simulink model "dsp48_firs_tb"  (Simulink 7.0)
settings: Solver=ode45  StartTime=0.0  StopTime=200  RelTol=1e-3
PreLoadFcn:
  | fir_setup_v1
StartFcn:
  | fir_setup_v1
undefined symbols (not defined in the file): A, B, C, coef, P, PCIN
libraries: xbsIndex_r4 x229, simulink x10, xbsCopyrightNotice_r4 x1, dspsrcs4 x1
(part 3 of 3)

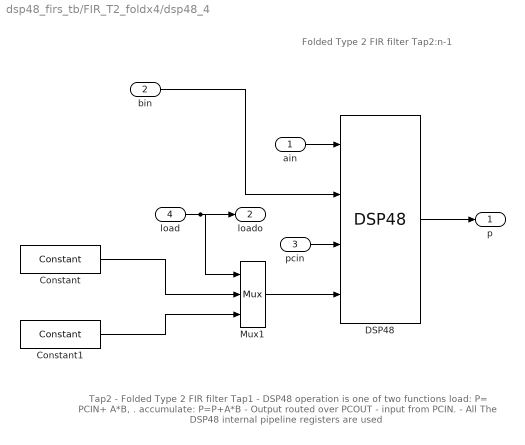
== system dsp48_firs_tb/FIR_T2_foldx4/dsp48_4 ==
  note: Folded Type 2 FIR filter Tap2:n-1
  note: Tap2 - Folded Type 2 FIR filter Tap1
      | - DSP48 operation is one of two functions
      |   load:  P= PCIN+ A*B, .
      |   accumulate: P=P+A*B
      | - Output routed over PCOUT
      | - input from PCIN.
      | - All The DSP48 internal pipeline registers are used
  ain : Inport  OutDataType=sfix(16)  OutScaling=2^0
  bin : Inport  Port=2  OutDataType=sfix(16)  OutScaling=2^0
  pcin : Inport  Port=3  OutDataType=sfix(16)  OutScaling=2^0
  load : Inport  Port=4  OutDataType=sfix(16)  OutScaling=2^0
  Constant : xbsIndex_r4/Constant  arith_type=DSP48 Instruction  const=1  n_bits=1  bin_pt=0  explicit_period=off  period=1  equ=P=P+(A*B)  opselect=P + A*B  inp2=PCIN>>17  opr=+  inp1=P  carry=CIN  dbl_ovrd=off  block_type=constant
      settings: block_version=VER_STRING_GOES_HERE
  Constant1 : xbsIndex_r4/Constant  arith_type=DSP48 Instruction  const=1  n_bits=1  bin_pt=0  explicit_period=off  period=1  equ=P=PCIN+(A*B)  opselect=PCIN + A*B  inp2=PCIN>>17  opr=+  inp1=P  carry=CIN  dbl_ovrd=off  block_type=constant
      settings: block_version=VER_STRING_GOES_HERE
  DSP48 : xbsIndex_r4/DSP48  use_b=Direct from B Port  use_op=on  use_creg=off  use_pcin=on  use_pcout=off  use_bcout=off  rst_all=off  en_all=off  pipeline_a=1  pipeline_b=1  pipeline_c=on  pipeline_p=on  pipeline_mult=on  pipeline_opmode=on  pipeline_sub=on  pipeline_carryin=on  pipeline_carryinsel=on  rst_a=off  rst_b=off  rst_c=off  rst_mult=off  rst_p=off  rst_carry_in=off  rst_ctrl=off  en_a=off  en_b=off  en_c=off  en_mult=off  en_p=off  en_carry_in=off  en_ctrl=off  dbl_ovrd=off  use_synth_model=off  xl_useadderonly=off  block_type=dsp48
      settings: xl_use_area=on  xl_area=[0, 0, 0, 0, 0, 0, 0]  block_version=VER_STRING_GOES_HERE
  Mux1 : xbsIndex_r4/Mux  inputs=2  en=off  latency=0  precision=Full  arith_type=Unsigned  n_bits=48  bin_pt=0  quantization=Truncate  overflow=Wrap  dbl_ovrd=off  block_type=mux
      settings: xl_area=[0, 0, 0, 0, 0, 0, 0]  block_version=VER_STRING_GOES_HERE
  p : Outport  OutDataType=sfix(16)  OutScaling=2^0
  loado : Outport  Port=2  OutDataType=sfix(16)  OutScaling=2^0
  wires:
  bin/1 -> DSP48/2
  ain/1 -> DSP48/1
  Constant1/1 -> Mux1/3
  Constant/1 -> Mux1/2
  load/1 -> loado/1, Mux1/1
  DSP48/1 -> p/1
  pcin/1 -> DSP48/3
  Mux1/1 -> DSP48/4

== system dsp48_firs_tb/FIR_T2x16 /fir_last ==
  note: Tapn- Parallel Type2 FIR filter
      | - DSP48 operation is the  function P=PCIN+ A*B.
      | - Input over PCIN, output is from P
      | - All The DSP48 internal pipeline registers are used
      | - The BCIN-BCOUT cascade is not used
  note: Parallel FIR Type2 Tap #n
  ain : Inport  OutDataType=sfix(16)  OutScaling=2^0
  bin : Inport  Port=2  OutDataType=sfix(16)  OutScaling=2^0
  pcin : Inport  Port=3  OutDataType=sfix(16)  OutScaling=2^0
  Constant1 : xbsIndex_r4/Constant  arith_type=DSP48 Instruction  const=1  n_bits=1  bin_pt=0  explicit_period=off  period=1  equ=P=PCIN+(A*B)  opselect=PCIN + A*B  inp2=PCIN>>17  opr=+  inp1=P  carry=CIN  dbl_ovrd=off  block_type=constant
      settings: block_version=VER_STRING_GOES_HERE
  DSP48 : xbsIndex_r4/DSP48  use_b=Direct from B Port  use_op=on  use_creg=off  use_pcin=on  use_pcout=off  use_bcout=off  rst_all=off  en_all=off  pipeline_a=1  pipeline_b=1  pipeline_c=on  pipeline_p=on  pipeline_mult=on  pipeline_opmode=on  pipeline_sub=on  pipeline_carryin=on  pipeline_carryinsel=on  rst_a=off  rst_b=off  rst_c=off  rst_mult=off  rst_p=off  rst_carry_in=off  rst_ctrl=off  en_a=off  en_b=off  en_c=off  en_mult=off  en_p=off  en_carry_in=off  en_ctrl=off  dbl_ovrd=off  use_synth_model=off  xl_useadderonly=off  block_type=dsp48
      settings: xl_use_area=on  xl_area=[0, 0, 0, 0, 0, 0, 0]  block_version=VER_STRING_GOES_HERE
  p : Outport  OutDataType=sfix(16)  OutScaling=2^0
  wires:
  bin/1 -> DSP48/2
  DSP48/1 -> p/1
  ain/1 -> DSP48/1
  pcin/1 -> DSP48/3
  Constant1/1 -> DSP48/4

== system dsp48_firs_tb/FIR_T2x16 /fir_next1 ==
  note: Tap2,n-1 - Parallel Type2 FIR filter
      | - DSP48 operation is the  function P=PCIN+ A*B.
      | - Input and Output routed over PCIN-PCOUT.
      | - All The DSP48 internal pipeline registers are used
      | - The BCIN-BCOUT cascade is not used
  note: Parallel FIR Type2 Tap #2:n-1
  ain : Inport  OutDataType=sfix(16)  OutScaling=2^0
  bin : Inport  Port=2  OutDataType=sfix(16)  OutScaling=2^0
  pcin : Inport  Port=3  OutDataType=sfix(16)  OutScaling=2^0
  Constant1 : xbsIndex_r4/Constant  arith_type=DSP48 Instruction  const=1  n_bits=1  bin_pt=0  explicit_period=off  period=1  equ=P=PCIN+(A*B)  opselect=PCIN + A*B  inp2=PCIN>>17  opr=+  inp1=P  carry=CIN  dbl_ovrd=off  block_type=constant
      settings: block_version=VER_STRING_GOES_HERE
  DSP48 : xbsIndex_r4/DSP48  use_b=Direct from B Port  use_op=on  use_creg=off  use_pcin=on  use_pcout=on  use_bcout=off  rst_all=off  en_all=off  pipeline_a=1  pipeline_b=1  pipeline_c=on  pipeline_p=on  pipeline_mult=on  pipeline_opmode=on  pipeline_sub=on  pipeline_carryin=on  pipeline_carryinsel=on  rst_a=off  rst_b=off  rst_c=off  rst_mult=off  rst_p=off  rst_carry_in=off  rst_ctrl=off  en_a=off  en_b=off  en_c=off  en_mult=off  en_p=off  en_carry_in=off  en_ctrl=off  dbl_ovrd=off  use_synth_model=off  xl_useadderonly=off  block_type=dsp48
      settings: xl_use_area=on  xl_area=[0, 0, 0, 0, 0, 0, 0]  block_version=VER_STRING_GOES_HERE
  Terminator1 : Terminator
  bout : Outport  OutDataType=sfix(16)  OutScaling=2^0
  pcout : Outport  Port=2  OutDataType=sfix(16)  OutScaling=2^0
  wires:
  bin/1 -> bout/1, DSP48/2
  ain/1 -> DSP48/1
  DSP48/2 -> pcout/1
  DSP48/1 -> Terminator1/1
  pcin/1 -> DSP48/3
  Constant1/1 -> DSP48/4

== system dsp48_firs_tb/FIR_T2x16 /fir_next10 ==
  note: Parallel FIR Type2 Tap #2:n-1
  note: Tap2,n-1 - Parallel Type2 FIR filter
      | - DSP48 operation is the  function P=PCIN+ A*B.
      | - Input and Output routed over PCIN-PCOUT.
      | - All The DSP48 internal pipeline registers are used
      | - The BCIN-BCOUT cascade is not used
  ain : Inport  OutDataType=sfix(16)  OutScaling=2^0
  bin : Inport  Port=2  OutDataType=sfix(16)  OutScaling=2^0
  pcin : Inport  Port=3  OutDataType=sfix(16)  OutScaling=2^0
  Constant1 : xbsIndex_r4/Constant  arith_type=DSP48 Instruction  const=1  n_bits=1  bin_pt=0  explicit_period=off  period=1  equ=P=PCIN+(A*B)  opselect=PCIN + A*B  inp2=PCIN>>17  opr=+  inp1=P  carry=CIN  dbl_ovrd=off  block_type=constant
      settings: block_version=VER_STRING_GOES_HERE
  DSP48 : xbsIndex_r4/DSP48  use_b=Direct from B Port  use_op=on  use_creg=off  use_pcin=on  use_pcout=on  use_bcout=off  rst_all=off  en_all=off  pipeline_a=1  pipeline_b=1  pipeline_c=on  pipeline_p=on  pipeline_mult=on  pipeline_opmode=on  pipeline_sub=on  pipeline_carryin=on  pipeline_carryinsel=on  rst_a=off  rst_b=off  rst_c=off  rst_mult=off  rst_p=off  rst_carry_in=off  rst_ctrl=off  en_a=off  en_b=off  en_c=off  en_mult=off  en_p=off  en_carry_in=off  en_ctrl=off  dbl_ovrd=off  use_synth_model=off  xl_useadderonly=off  block_type=dsp48
      settings: xl_use_area=on  xl_area=[0, 0, 0, 0, 0, 0, 0]  block_version=VER_STRING_GOES_HERE
  Terminator1 : Terminator
  bout : Outport  OutDataType=sfix(16)  OutScaling=2^0
  pcout : Outport  Port=2  OutDataType=sfix(16)  OutScaling=2^0
  wires:
  Constant1/1 -> DSP48/4
  pcin/1 -> DSP48/3
  DSP48/1 -> Terminator1/1
  DSP48/2 -> pcout/1
  ain/1 -> DSP48/1
  bin/1 -> DSP48/2, bout/1

== system dsp48_firs_tb/FIR_T2x16 /fir_next11 ==
  note: Tap2,n-1 - Parallel Type2 FIR filter
      | - DSP48 operation is the  function P=PCIN+ A*B.
      | - Input and Output routed over PCIN-PCOUT.
      | - All The DSP48 internal pipeline registers are used
      | - The BCIN-BCOUT cascade is not used
  note: Parallel FIR Type2 Tap #2:n-1
  ain : Inport  OutDataType=sfix(16)  OutScaling=2^0
  bin : Inport  Port=2  OutDataType=sfix(16)  OutScaling=2^0
  pcin : Inport  Port=3  OutDataType=sfix(16)  OutScaling=2^0
  Constant1 : xbsIndex_r4/Constant  arith_type=DSP48 Instruction  const=1  n_bits=1  bin_pt=0  explicit_period=off  period=1  equ=P=PCIN+(A*B)  opselect=PCIN + A*B  inp2=PCIN>>17  opr=+  inp1=P  carry=CIN  dbl_ovrd=off  block_type=constant
      settings: block_version=VER_STRING_GOES_HERE
  DSP48 : xbsIndex_r4/DSP48  use_b=Direct from B Port  use_op=on  use_creg=off  use_pcin=on  use_pcout=on  use_bcout=off  rst_all=off  en_all=off  pipeline_a=1  pipeline_b=1  pipeline_c=on  pipeline_p=on  pipeline_mult=on  pipeline_opmode=on  pipeline_sub=on  pipeline_carryin=on  pipeline_carryinsel=on  rst_a=off  rst_b=off  rst_c=off  rst_mult=off  rst_p=off  rst_carry_in=off  rst_ctrl=off  en_a=off  en_b=off  en_c=off  en_mult=off  en_p=off  en_carry_in=off  en_ctrl=off  dbl_ovrd=off  use_synth_model=off  xl_useadderonly=off  block_type=dsp48
      settings: xl_use_area=on  xl_area=[0, 0, 0, 0, 0, 0, 0]  block_version=VER_STRING_GOES_HERE
  Terminator1 : Terminator
  bout : Outport  OutDataType=sfix(16)  OutScaling=2^0
  pcout : Outport  Port=2  OutDataType=sfix(16)  OutScaling=2^0
  wires:
  bin/1 -> bout/1, DSP48/2
  ain/1 -> DSP48/1
  DSP48/2 -> pcout/1
  DSP48/1 -> Terminator1/1
  pcin/1 -> DSP48/3
  Constant1/1 -> DSP48/4

== system dsp48_firs_tb/FIR_T2x16 /fir_next12 ==
  note: Parallel FIR Type2 Tap #2:n-1
  note: Tap2,n-1 - Parallel Type2 FIR filter
      | - DSP48 operation is the  function P=PCIN+ A*B.
      | - Input and Output routed over PCIN-PCOUT.
      | - All The DSP48 internal pipeline registers are used
      | - The BCIN-BCOUT cascade is not used
  ain : Inport  OutDataType=sfix(16)  OutScaling=2^0
  bin : Inport  Port=2  OutDataType=sfix(16)  OutScaling=2^0
  pcin : Inport  Port=3  OutDataType=sfix(16)  OutScaling=2^0
  Constant1 : xbsIndex_r4/Constant  arith_type=DSP48 Instruction  const=1  n_bits=1  bin_pt=0  explicit_period=off  period=1  equ=P=PCIN+(A*B)  opselect=PCIN + A*B  inp2=PCIN>>17  opr=+  inp1=P  carry=CIN  dbl_ovrd=off  block_type=constant
      settings: block_version=VER_STRING_GOES_HERE
  DSP48 : xbsIndex_r4/DSP48  use_b=Direct from B Port  use_op=on  use_creg=off  use_pcin=on  use_pcout=on  use_bcout=off  rst_all=off  en_all=off  pipeline_a=1  pipeline_b=1  pipeline_c=on  pipeline_p=on  pipeline_mult=on  pipeline_opmode=on  pipeline_sub=on  pipeline_carryin=on  pipeline_carryinsel=on  rst_a=off  rst_b=off  rst_c=off  rst_mult=off  rst_p=off  rst_carry_in=off  rst_ctrl=off  en_a=off  en_b=off  en_c=off  en_mult=off  en_p=off  en_carry_in=off  en_ctrl=off  dbl_ovrd=off  use_synth_model=off  xl_useadderonly=off  block_type=dsp48
      settings: xl_use_area=on  xl_area=[0, 0, 0, 0, 0, 0, 0]  block_version=VER_STRING_GOES_HERE
  Terminator1 : Terminator
  bout : Outport  OutDataType=sfix(16)  OutScaling=2^0
  pcout : Outport  Port=2  OutDataType=sfix(16)  OutScaling=2^0
  wires:
  Constant1/1 -> DSP48/4
  pcin/1 -> DSP48/3
  DSP48/1 -> Terminator1/1
  DSP48/2 -> pcout/1
  ain/1 -> DSP48/1
  bin/1 -> DSP48/2, bout/1

== system dsp48_firs_tb/FIR_T2x16 /fir_next13 ==
  note: Tap2,n-1 - Parallel Type2 FIR filter
      | - DSP48 operation is the  function P=PCIN+ A*B.
      | - Input and Output routed over PCIN-PCOUT.
      | - All The DSP48 internal pipeline registers are used
      | - The BCIN-BCOUT cascade is not used
  note: Parallel FIR Type2 Tap #2:n-1
  ain : Inport  OutDataType=sfix(16)  OutScaling=2^0
  bin : Inport  Port=2  OutDataType=sfix(16)  OutScaling=2^0
  pcin : Inport  Port=3  OutDataType=sfix(16)  OutScaling=2^0
  Constant1 : xbsIndex_r4/Constant  arith_type=DSP48 Instruction  const=1  n_bits=1  bin_pt=0  explicit_period=off  period=1  equ=P=PCIN+(A*B)  opselect=PCIN + A*B  inp2=PCIN>>17  opr=+  inp1=P  carry=CIN  dbl_ovrd=off  block_type=constant
      settings: block_version=VER_STRING_GOES_HERE
  DSP48 : xbsIndex_r4/DSP48  use_b=Direct from B Port  use_op=on  use_creg=off  use_pcin=on  use_pcout=on  use_bcout=off  rst_all=off  en_all=off  pipeline_a=1  pipeline_b=1  pipeline_c=on  pipeline_p=on  pipeline_mult=on  pipeline_opmode=on  pipeline_sub=on  pipeline_carryin=on  pipeline_carryinsel=on  rst_a=off  rst_b=off  rst_c=off  rst_mult=off  rst_p=off  rst_carry_in=off  rst_ctrl=off  en_a=off  en_b=off  en_c=off  en_mult=off  en_p=off  en_carry_in=off  en_ctrl=off  dbl_ovrd=off  use_synth_model=off  xl_useadderonly=off  block_type=dsp48
      settings: xl_use_area=on  xl_area=[0, 0, 0, 0, 0, 0, 0]  block_version=VER_STRING_GOES_HERE
  Terminator1 : Terminator
  bout : Outport  OutDataType=sfix(16)  OutScaling=2^0
  pcout : Outport  Port=2  OutDataType=sfix(16)  OutScaling=2^0
  wires:
  bin/1 -> bout/1, DSP48/2
  ain/1 -> DSP48/1
  DSP48/2 -> pcout/1
  DSP48/1 -> Terminator1/1
  pcin/1 -> DSP48/3
  Constant1/1 -> DSP48/4

== system dsp48_firs_tb/FIR_T2x16 /fir_next14 ==
  note: Parallel FIR Type2 Tap #2:n-1
  note: Tap2,n-1 - Parallel Type2 FIR filter
      | - DSP48 operation is the  function P=PCIN+ A*B.
      | - Input and Output routed over PCIN-PCOUT.
      | - All The DSP48 internal pipeline registers are used
      | - The BCIN-BCOUT cascade is not used
  ain : Inport  OutDataType=sfix(16)  OutScaling=2^0
  bin : Inport  Port=2  OutDataType=sfix(16)  OutScaling=2^0
  pcin : Inport  Port=3  OutDataType=sfix(16)  OutScaling=2^0
  Constant1 : xbsIndex_r4/Constant  arith_type=DSP48 Instruction  const=1  n_bits=1  bin_pt=0  explicit_period=off  period=1  equ=P=PCIN+(A*B)  opselect=PCIN + A*B  inp2=PCIN>>17  opr=+  inp1=P  carry=CIN  dbl_ovrd=off  block_type=constant
      settings: block_version=VER_STRING_GOES_HERE
  DSP48 : xbsIndex_r4/DSP48  use_b=Direct from B Port  use_op=on  use_creg=off  use_pcin=on  use_pcout=on  use_bcout=off  rst_all=off  en_all=off  pipeline_a=1  pipeline_b=1  pipeline_c=on  pipeline_p=on  pipeline_mult=on  pipeline_opmode=on  pipeline_sub=on  pipeline_carryin=on  pipeline_carryinsel=on  rst_a=off  rst_b=off  rst_c=off  rst_mult=off  rst_p=off  rst_carry_in=off  rst_ctrl=off  en_a=off  en_b=off  en_c=off  en_mult=off  en_p=off  en_carry_in=off  en_ctrl=off  dbl_ovrd=off  use_synth_model=off  xl_useadderonly=off  block_type=dsp48
      settings: xl_use_area=on  xl_area=[0, 0, 0, 0, 0, 0, 0]  block_version=VER_STRING_GOES_HERE
  Terminator1 : Terminator
  bout : Outport  OutDataType=sfix(16)  OutScaling=2^0
  pcout : Outport  Port=2  OutDataType=sfix(16)  OutScaling=2^0
  wires:
  Constant1/1 -> DSP48/4
  pcin/1 -> DSP48/3
  DSP48/1 -> Terminator1/1
  DSP48/2 -> pcout/1
  ain/1 -> DSP48/1
  bin/1 -> DSP48/2, bout/1

== system dsp48_firs_tb/FIR_T2x16 /fir_next2 ==
  note: Parallel FIR Type2 Tap #2:n-1
  note: Tap2,n-1 - Parallel Type2 FIR filter
      | - DSP48 operation is the  function P=PCIN+ A*B.
      | - Input and Output routed over PCIN-PCOUT.
      | - All The DSP48 internal pipeline registers are used
      | - The BCIN-BCOUT cascade is not used
  ain : Inport  OutDataType=sfix(16)  OutScaling=2^0
  bin : Inport  Port=2  OutDataType=sfix(16)  OutScaling=2^0
  pcin : Inport  Port=3  OutDataType=sfix(16)  OutScaling=2^0
  Constant1 : xbsIndex_r4/Constant  arith_type=DSP48 Instruction  const=1  n_bits=1  bin_pt=0  explicit_period=off  period=1  equ=P=PCIN+(A*B)  opselect=PCIN + A*B  inp2=PCIN>>17  opr=+  inp1=P  carry=CIN  dbl_ovrd=off  block_type=constant
      settings: block_version=VER_STRING_GOES_HERE
  DSP48 : xbsIndex_r4/DSP48  use_b=Direct from B Port  use_op=on  use_creg=off  use_pcin=on  use_pcout=on  use_bcout=off  rst_all=off  en_all=off  pipeline_a=1  pipeline_b=1  pipeline_c=on  pipeline_p=on  pipeline_mult=on  pipeline_opmode=on  pipeline_sub=on  pipeline_carryin=on  pipeline_carryinsel=on  rst_a=off  rst_b=off  rst_c=off  rst_mult=off  rst_p=off  rst_carry_in=off  rst_ctrl=off  en_a=off  en_b=off  en_c=off  en_mult=off  en_p=off  en_carry_in=off  en_ctrl=off  dbl_ovrd=off  use_synth_model=off  xl_useadderonly=off  block_type=dsp48
      settings: xl_use_area=on  xl_area=[0, 0, 0, 0, 0, 0, 0]  block_version=VER_STRING_GOES_HERE
  Terminator1 : Terminator
  bout : Outport  OutDataType=sfix(16)  OutScaling=2^0
  pcout : Outport  Port=2  OutDataType=sfix(16)  OutScaling=2^0
  wires:
  Constant1/1 -> DSP48/4
  pcin/1 -> DSP48/3
  DSP48/1 -> Terminator1/1
  DSP48/2 -> pcout/1
  ain/1 -> DSP48/1
  bin/1 -> DSP48/2, bout/1

== system dsp48_firs_tb/FIR_T2x16 /fir_next3 ==
  note: Tap2,n-1 - Parallel Type2 FIR filter
      | - DSP48 operation is the  function P=PCIN+ A*B.
      | - Input and Output routed over PCIN-PCOUT.
      | - All The DSP48 internal pipeline registers are used
      | - The BCIN-BCOUT cascade is not used
  note: Parallel FIR Type2 Tap #2:n-1
  ain : Inport  OutDataType=sfix(16)  OutScaling=2^0
  bin : Inport  Port=2  OutDataType=sfix(16)  OutScaling=2^0
  pcin : Inport  Port=3  OutDataType=sfix(16)  OutScaling=2^0
  Constant1 : xbsIndex_r4/Constant  arith_type=DSP48 Instruction  const=1  n_bits=1  bin_pt=0  explicit_period=off  period=1  equ=P=PCIN+(A*B)  opselect=PCIN + A*B  inp2=PCIN>>17  opr=+  inp1=P  carry=CIN  dbl_ovrd=off  block_type=constant
      settings: block_version=VER_STRING_GOES_HERE
  DSP48 : xbsIndex_r4/DSP48  use_b=Direct from B Port  use_op=on  use_creg=off  use_pcin=on  use_pcout=on  use_bcout=off  rst_all=off  en_all=off  pipeline_a=1  pipeline_b=1  pipeline_c=on  pipeline_p=on  pipeline_mult=on  pipeline_opmode=on  pipeline_sub=on  pipeline_carryin=on  pipeline_carryinsel=on  rst_a=off  rst_b=off  rst_c=off  rst_mult=off  rst_p=off  rst_carry_in=off  rst_ctrl=off  en_a=off  en_b=off  en_c=off  en_mult=off  en_p=off  en_carry_in=off  en_ctrl=off  dbl_ovrd=off  use_synth_model=off  xl_useadderonly=off  block_type=dsp48
      settings: xl_use_area=on  xl_area=[0, 0, 0, 0, 0, 0, 0]  block_version=VER_STRING_GOES_HERE
  Terminator1 : Terminator
  bout : Outport  OutDataType=sfix(16)  OutScaling=2^0
  pcout : Outport  Port=2  OutDataType=sfix(16)  OutScaling=2^0
  wires:
  bin/1 -> bout/1, DSP48/2
  ain/1 -> DSP48/1
  DSP48/2 -> pcout/1
  DSP48/1 -> Terminator1/1
  pcin/1 -> DSP48/3
  Constant1/1 -> DSP48/4

== system dsp48_firs_tb/FIR_T2x16 /fir_next4 ==
  note: Parallel FIR Type2 Tap #2:n-1
  note: Tap2,n-1 - Parallel Type2 FIR filter
      | - DSP48 operation is the  function P=PCIN+ A*B.
      | - Input and Output routed over PCIN-PCOUT.
      | - All The DSP48 internal pipeline registers are used
      | - The BCIN-BCOUT cascade is not used
  ain : Inport  OutDataType=sfix(16)  OutScaling=2^0
  bin : Inport  Port=2  OutDataType=sfix(16)  OutScaling=2^0
  pcin : Inport  Port=3  OutDataType=sfix(16)  OutScaling=2^0
  Constant1 : xbsIndex_r4/Constant  arith_type=DSP48 Instruction  const=1  n_bits=1  bin_pt=0  explicit_period=off  period=1  equ=P=PCIN+(A*B)  opselect=PCIN + A*B  inp2=PCIN>>17  opr=+  inp1=P  carry=CIN  dbl_ovrd=off  block_type=constant
      settings: block_version=VER_STRING_GOES_HERE
  DSP48 : xbsIndex_r4/DSP48  use_b=Direct from B Port  use_op=on  use_creg=off  use_pcin=on  use_pcout=on  use_bcout=off  rst_all=off  en_all=off  pipeline_a=1  pipeline_b=1  pipeline_c=on  pipeline_p=on  pipeline_mult=on  pipeline_opmode=on  pipeline_sub=on  pipeline_carryin=on  pipeline_carryinsel=on  rst_a=off  rst_b=off  rst_c=off  rst_mult=off  rst_p=off  rst_carry_in=off  rst_ctrl=off  en_a=off  en_b=off  en_c=off  en_mult=off  en_p=off  en_carry_in=off  en_ctrl=off  dbl_ovrd=off  use_synth_model=off  xl_useadderonly=off  block_type=dsp48
      settings: xl_use_area=on  xl_area=[0, 0, 0, 0, 0, 0, 0]  block_version=VER_STRING_GOES_HERE
  Terminator1 : Terminator
  bout : Outport  OutDataType=sfix(16)  OutScaling=2^0
  pcout : Outport  Port=2  OutDataType=sfix(16)  OutScaling=2^0
  wires:
  Constant1/1 -> DSP48/4
  pcin/1 -> DSP48/3
  DSP48/1 -> Terminator1/1
  DSP48/2 -> pcout/1
  ain/1 -> DSP48/1
  bin/1 -> DSP48/2, bout/1

== system dsp48_firs_tb/FIR_T2x16 /fir_next5 ==
  note: Tap2,n-1 - Parallel Type2 FIR filter
      | - DSP48 operation is the  function P=PCIN+ A*B.
      | - Input and Output routed over PCIN-PCOUT.
      | - All The DSP48 internal pipeline registers are used
      | - The BCIN-BCOUT cascade is not used
  note: Parallel FIR Type2 Tap #2:n-1
  ain : Inport  OutDataType=sfix(16)  OutScaling=2^0
  bin : Inport  Port=2  OutDataType=sfix(16)  OutScaling=2^0
  pcin : Inport  Port=3  OutDataType=sfix(16)  OutScaling=2^0
  Constant1 : xbsIndex_r4/Constant  arith_type=DSP48 Instruction  const=1  n_bits=1  bin_pt=0  explicit_period=off  period=1  equ=P=PCIN+(A*B)  opselect=PCIN + A*B  inp2=PCIN>>17  opr=+  inp1=P  carry=CIN  dbl_ovrd=off  block_type=constant
      settings: block_version=VER_STRING_GOES_HERE
  DSP48 : xbsIndex_r4/DSP48  use_b=Direct from B Port  use_op=on  use_creg=off  use_pcin=on  use_pcout=on  use_bcout=off  rst_all=off  en_all=off  pipeline_a=1  pipeline_b=1  pipeline_c=on  pipeline_p=on  pipeline_mult=on  pipeline_opmode=on  pipeline_sub=on  pipeline_carryin=on  pipeline_carryinsel=on  rst_a=off  rst_b=off  rst_c=off  rst_mult=off  rst_p=off  rst_carry_in=off  rst_ctrl=off  en_a=off  en_b=off  en_c=off  en_mult=off  en_p=off  en_carry_in=off  en_ctrl=off  dbl_ovrd=off  use_synth_model=off  xl_useadderonly=off  block_type=dsp48
      settings: xl_use_area=on  xl_area=[0, 0, 0, 0, 0, 0, 0]  block_version=VER_STRING_GOES_HERE
  Terminator1 : Terminator
  bout : Outport  OutDataType=sfix(16)  OutScaling=2^0
  pcout : Outport  Port=2  OutDataType=sfix(16)  OutScaling=2^0
  wires:
  bin/1 -> bout/1, DSP48/2
  ain/1 -> DSP48/1
  DSP48/2 -> pcout/1
  DSP48/1 -> Terminator1/1
  pcin/1 -> DSP48/3
  Constant1/1 -> DSP48/4

== system dsp48_firs_tb/FIR_T2x16 /fir_next6 ==
  note: Parallel FIR Type2 Tap #2:n-1
  note: Tap2,n-1 - Parallel Type2 FIR filter
      | - DSP48 operation is the  function P=PCIN+ A*B.
      | - Input and Output routed over PCIN-PCOUT.
      | - All The DSP48 internal pipeline registers are used
      | - The BCIN-BCOUT cascade is not used
  ain : Inport  OutDataType=sfix(16)  OutScaling=2^0
  bin : Inport  Port=2  OutDataType=sfix(16)  OutScaling=2^0
  pcin : Inport  Port=3  OutDataType=sfix(16)  OutScaling=2^0
  Constant1 : xbsIndex_r4/Constant  arith_type=DSP48 Instruction  const=1  n_bits=1  bin_pt=0  explicit_period=off  period=1  equ=P=PCIN+(A*B)  opselect=PCIN + A*B  inp2=PCIN>>17  opr=+  inp1=P  carry=CIN  dbl_ovrd=off  block_type=constant
      settings: block_version=VER_STRING_GOES_HERE
  DSP48 : xbsIndex_r4/DSP48  use_b=Direct from B Port  use_op=on  use_creg=off  use_pcin=on  use_pcout=on  use_bcout=off  rst_all=off  en_all=off  pipeline_a=1  pipeline_b=1  pipeline_c=on  pipeline_p=on  pipeline_mult=on  pipeline_opmode=on  pipeline_sub=on  pipeline_carryin=on  pipeline_carryinsel=on  rst_a=off  rst_b=off  rst_c=off  rst_mult=off  rst_p=off  rst_carry_in=off  rst_ctrl=off  en_a=off  en_b=off  en_c=off  en_mult=off  en_p=off  en_carry_in=off  en_ctrl=off  dbl_ovrd=off  use_synth_model=off  xl_useadderonly=off  block_type=dsp48
      settings: xl_use_area=on  xl_area=[0, 0, 0, 0, 0, 0, 0]  block_version=VER_STRING_GOES_HERE
  Terminator1 : Terminator
  bout : Outport  OutDataType=sfix(16)  OutScaling=2^0
  pcout : Outport  Port=2  OutDataType=sfix(16)  OutScaling=2^0
  wires:
  Constant1/1 -> DSP48/4
  pcin/1 -> DSP48/3
  DSP48/1 -> Terminator1/1
  DSP48/2 -> pcout/1
  ain/1 -> DSP48/1
  bin/1 -> DSP48/2, bout/1

== system dsp48_firs_tb/FIR_T2x16 /fir_next7 ==
  note: Tap2,n-1 - Parallel Type2 FIR filter
      | - DSP48 operation is the  function P=PCIN+ A*B.
      | - Input and Output routed over PCIN-PCOUT.
      | - All The DSP48 internal pipeline registers are used
      | - The BCIN-BCOUT cascade is not used
  note: Parallel FIR Type2 Tap #2:n-1
  ain : Inport  OutDataType=sfix(16)  OutScaling=2^0
  bin : Inport  Port=2  OutDataType=sfix(16)  OutScaling=2^0
  pcin : Inport  Port=3  OutDataType=sfix(16)  OutScaling=2^0
  Constant1 : xbsIndex_r4/Constant  arith_type=DSP48 Instruction  const=1  n_bits=1  bin_pt=0  explicit_period=off  period=1  equ=P=PCIN+(A*B)  opselect=PCIN + A*B  inp2=PCIN>>17  opr=+  inp1=P  carry=CIN  dbl_ovrd=off  block_type=constant
      settings: block_version=VER_STRING_GOES_HERE
  DSP48 : xbsIndex_r4/DSP48  use_b=Direct from B Port  use_op=on  use_creg=off  use_pcin=on  use_pcout=on  use_bcout=off  rst_all=off  en_all=off  pipeline_a=1  pipeline_b=1  pipeline_c=on  pipeline_p=on  pipeline_mult=on  pipeline_opmode=on  pipeline_sub=on  pipeline_carryin=on  pipeline_carryinsel=on  rst_a=off  rst_b=off  rst_c=off  rst_mult=off  rst_p=off  rst_carry_in=off  rst_ctrl=off  en_a=off  en_b=off  en_c=off  en_mult=off  en_p=off  en_carry_in=off  en_ctrl=off  dbl_ovrd=off  use_synth_model=off  xl_useadderonly=off  block_type=dsp48
      settings: xl_use_area=on  xl_area=[0, 0, 0, 0, 0, 0, 0]  block_version=VER_STRING_GOES_HERE
  Terminator1 : Terminator
  bout : Outport  OutDataType=sfix(16)  OutScaling=2^0
  pcout : Outport  Port=2  OutDataType=sfix(16)  OutScaling=2^0
  wires:
  bin/1 -> bout/1, DSP48/2
  ain/1 -> DSP48/1
  DSP48/2 -> pcout/1
  DSP48/1 -> Terminator1/1
  pcin/1 -> DSP48/3
  Constant1/1 -> DSP48/4

== system dsp48_firs_tb/FIR_T2x16 /fir_next8 ==
  note: Parallel FIR Type2 Tap #2:n-1
  note: Tap2,n-1 - Parallel Type2 FIR filter
      | - DSP48 operation is the  function P=PCIN+ A*B.
      | - Input and Output routed over PCIN-PCOUT.
      | - All The DSP48 internal pipeline registers are used
      | - The BCIN-BCOUT cascade is not used
  ain : Inport  OutDataType=sfix(16)  OutScaling=2^0
  bin : Inport  Port=2  OutDataType=sfix(16)  OutScaling=2^0
  pcin : Inport  Port=3  OutDataType=sfix(16)  OutScaling=2^0
  Constant1 : xbsIndex_r4/Constant  arith_type=DSP48 Instruction  const=1  n_bits=1  bin_pt=0  explicit_period=off  period=1  equ=P=PCIN+(A*B)  opselect=PCIN + A*B  inp2=PCIN>>17  opr=+  inp1=P  carry=CIN  dbl_ovrd=off  block_type=constant
      settings: block_version=VER_STRING_GOES_HERE
  DSP48 : xbsIndex_r4/DSP48  use_b=Direct from B Port  use_op=on  use_creg=off  use_pcin=on  use_pcout=on  use_bcout=off  rst_all=off  en_all=off  pipeline_a=1  pipeline_b=1  pipeline_c=on  pipeline_p=on  pipeline_mult=on  pipeline_opmode=on  pipeline_sub=on  pipeline_carryin=on  pipeline_carryinsel=on  rst_a=off  rst_b=off  rst_c=off  rst_mult=off  rst_p=off  rst_carry_in=off  rst_ctrl=off  en_a=off  en_b=off  en_c=off  en_mult=off  en_p=off  en_carry_in=off  en_ctrl=off  dbl_ovrd=off  use_synth_model=off  xl_useadderonly=off  block_type=dsp48
      settings: xl_use_area=on  xl_area=[0, 0, 0, 0, 0, 0, 0]  block_version=VER_STRING_GOES_HERE
  Terminator1 : Terminator
  bout : Outport  OutDataType=sfix(16)  OutScaling=2^0
  pcout : Outport  Port=2  OutDataType=sfix(16)  OutScaling=2^0
  wires:
  Constant1/1 -> DSP48/4
  pcin/1 -> DSP48/3
  DSP48/1 -> Terminator1/1
  DSP48/2 -> pcout/1
  ain/1 -> DSP48/1
  bin/1 -> DSP48/2, bout/1

== system dsp48_firs_tb/FIR_T2x16 /fir_next9 ==
  note: Tap2,n-1 - Parallel Type2 FIR filter
      | - DSP48 operation is the  function P=PCIN+ A*B.
      | - Input and Output routed over PCIN-PCOUT.
      | - All The DSP48 internal pipeline registers are used
      | - The BCIN-BCOUT cascade is not used
  note: Parallel FIR Type2 Tap #2:n-1
  ain : Inport  OutDataType=sfix(16)  OutScaling=2^0
  bin : Inport  Port=2  OutDataType=sfix(16)  OutScaling=2^0
  pcin : Inport  Port=3  OutDataType=sfix(16)  OutScaling=2^0
  Constant1 : xbsIndex_r4/Constant  arith_type=DSP48 Instruction  const=1  n_bits=1  bin_pt=0  explicit_period=off  period=1  equ=P=PCIN+(A*B)  opselect=PCIN + A*B  inp2=PCIN>>17  opr=+  inp1=P  carry=CIN  dbl_ovrd=off  block_type=constant
      settings: block_version=VER_STRING_GOES_HERE
  DSP48 : xbsIndex_r4/DSP48  use_b=Direct from B Port  use_op=on  use_creg=off  use_pcin=on  use_pcout=on  use_bcout=off  rst_all=off  en_all=off  pipeline_a=1  pipeline_b=1  pipeline_c=on  pipeline_p=on  pipeline_mult=on  pipeline_opmode=on  pipeline_sub=on  pipeline_carryin=on  pipeline_carryinsel=on  rst_a=off  rst_b=off  rst_c=off  rst_mult=off  rst_p=off  rst_carry_in=off  rst_ctrl=off  en_a=off  en_b=off  en_c=off  en_mult=off  en_p=off  en_carry_in=off  en_ctrl=off  dbl_ovrd=off  use_synth_model=off  xl_useadderonly=off  block_type=dsp48
      settings: xl_use_area=on  xl_area=[0, 0, 0, 0, 0, 0, 0]  block_version=VER_STRING_GOES_HERE
  Terminator1 : Terminator
  bout : Outport  OutDataType=sfix(16)  OutScaling=2^0
  pcout : Outport  Port=2  OutDataType=sfix(16)  OutScaling=2^0
  wires:
  bin/1 -> bout/1, DSP48/2
  ain/1 -> DSP48/1
  DSP48/2 -> pcout/1
  DSP48/1 -> Terminator1/1
  pcin/1 -> DSP48/3
  Constant1/1 -> DSP48/4

== system dsp48_firs_tb/FIR_T2x16 /fir_start ==
  note: Parallel FIR Type2 Tap #1
  note: Tap1 - Parallel Type2 FIR filter
      | - DSP48 operation is the  function P=C+ A*B.
      | - Output routed over PCOUT.
      | - All The DSP48 internal pipeline registers are used
      | - The BCIN-BCOUT cascade is not used
  ain : Inport  OutDataType=sfix(16)  OutScaling=2^0
  bin : Inport  Port=2  OutDataType=sfix(16)  OutScaling=2^0
  c : Inport  Port=3  OutDataType=sfix(16)  OutScaling=2^0
  Constant : xbsIndex_r4/Constant  arith_type=DSP48 Instruction  const=1  n_bits=1  bin_pt=0  explicit_period=off  period=1  equ=P=C+(A*B)  opselect=C + A*B  inp2=PCIN>>17  opr=+  inp1=P  carry=CIN  dbl_ovrd=off  block_type=constant
      settings: block_version=VER_STRING_GOES_HERE
  DSP48 : xbsIndex_r4/DSP48  use_b=Direct from B Port  use_op=on  use_creg=on  use_pcin=off  use_pcout=on  use_bcout=off  rst_all=off  en_all=off  pipeline_a=1  pipeline_b=1  pipeline_c=on  pipeline_p=on  pipeline_mult=on  pipeline_opmode=on  pipeline_sub=on  pipeline_carryin=on  pipeline_carryinsel=on  rst_a=off  rst_b=off  rst_c=off  rst_mult=off  rst_p=off  rst_carry_in=off  rst_ctrl=off  en_a=off  en_b=off  en_c=off  en_mult=off  en_p=off  en_carry_in=off  en_ctrl=off  dbl_ovrd=off  use_synth_model=off  xl_useadderonly=off  block_type=dsp48
      settings: xl_use_area=on  xl_area=[0, 0, 0, 0, 0, 0, 0]  block_version=VER_STRING_GOES_HERE
  Terminator1 : Terminator
  bout : Outport  OutDataType=sfix(16)  OutScaling=2^0
  pcout : Outport  Port=2  OutDataType=sfix(16)  OutScaling=2^0
  wires:
  Constant/1 -> DSP48/4
  ain/1 -> DSP48/1
  c/1 -> DSP48/3
  bin/1 -> DSP48/2, bout/1
  DSP48/2 -> pcout/1
  DSP48/1 -> Terminator1/1

== system dsp48_firs_tb/FIR_foldx16/dsp48 ==
  note: Multiply Accumulate (MAC)
  note: MAC - Multiply Accumulate Block
      | - DSP48 operation is one of two functions
      |   load:  P= A*B, .
      |   accumulate: P=P+A*B
      | - Output routed over P.
      | - All The DSP48 internal pipeline registers are used
  ain : Inport  OutDataType=sfix(16)  OutScaling=2^0
  bin : Inport  Port=2  OutDataType=sfix(16)  OutScaling=2^0
  c : Inport  Port=3  OutDataType=sfix(16)  OutScaling=2^0
  load : Inport  Port=4  OutDataType=sfix(16)  OutScaling=2^0
  Constant : xbsIndex_r4/Constant  arith_type=DSP48 Instruction  const=1  n_bits=1  bin_pt=0  explicit_period=off  period=1  equ=P=P+(A*B)  opselect=P + A*B  inp2=PCIN>>17  opr=+  inp1=P  carry=CIN  dbl_ovrd=off  block_type=constant
      settings: block_version=VER_STRING_GOES_HERE
  Constant1 : xbsIndex_r4/Constant  arith_type=DSP48 Instruction  const=1  n_bits=1  bin_pt=0  explicit_period=off  period=1  equ=P=+A*B  opselect=A * B  inp2=PCIN>>17  opr=+  inp1=P  carry=CIN  dbl_ovrd=off  block_type=constant
      settings: block_version=VER_STRING_GOES_HERE
  DSP48 : xbsIndex_r4/DSP48  use_b=Direct from B Port  use_op=on  use_creg=on  use_pcin=off  use_pcout=off  use_bcout=off  rst_all=off  en_all=off  pipeline_a=1  pipeline_b=1  pipeline_c=on  pipeline_p=on  pipeline_mult=on  pipeline_opmode=on  pipeline_sub=on  pipeline_carryin=on  pipeline_carryinsel=on  rst_a=off  rst_b=off  rst_c=off  rst_mult=off  rst_p=off  rst_carry_in=off  rst_ctrl=off  en_a=off  en_b=off  en_c=off  en_mult=off  en_p=off  en_carry_in=off  en_ctrl=off  dbl_ovrd=off  use_synth_model=off  xl_useadderonly=off  block_type=dsp48
      settings: xl_use_area=on  xl_area=[0, 0, 0, 0, 0, 0, 0]  block_version=VER_STRING_GOES_HERE
  Mux1 : xbsIndex_r4/Mux  inputs=2  en=off  latency=0  precision=Full  arith_type=Unsigned  n_bits=48  bin_pt=0  quantization=Truncate  overflow=Wrap  dbl_ovrd=off  block_type=mux
      settings: xl_area=[0, 0, 0, 0, 0, 0, 0]  block_version=VER_STRING_GOES_HERE
  out : Outport  OutDataType=sfix(16)  OutScaling=2^0
  wires:
  c/1 -> DSP48/3
  bin/1 -> DSP48/2
  ain/1 -> DSP48/1
  DSP48/1 -> out/1
  Mux1/1 -> DSP48/4
  load/1 -> Mux1/1
  Constant1/1 -> Mux1/3
  Constant/1 -> Mux1/2
